simulink model "SecRwLtStZeroCtrl"  (R2018b)
settings: Solver=FixedStepDiscrete  StartTime=0.0  StopTime=10.0  RelTol=1e-3
undefined symbols (not defined in the file or in its folder): KeSMSuMdMotFinshdTm_Val, KeSMSuMdRetryTm1_Val, KeSMSuModeReqDurgTm_Val, KeSMSwSecRwLtStZeroEnTrigBitMask_Val
libraries: StCtrlLibBkRecln x1
settings Model: Creator=sn2xws  LastModifiedBy=sn55gm
settings Model: ModifiedHistory=|
  | 2024.5.6
  | 557 First Release
  | 2024.8.14 bitmask更换为port接口
settings DataIOCC: SaveFormat=StructureWithTime
settings OptimizationCC: DefaultParameterBehavior=Inlined  EnhancedBackFolding=on  PassReuseOutputArgsAs=Individual arguments  ZeroExternalMemoryAtStartup=off  ZeroInternalMemoryAtStartup=off  OptimizeBlockOrder=speed  DifferentSizesBufferReuse=on  OptimizationCustomize=off
settings DebuggingCC: ParameterTunabilityLossMsg=error
settings SFSimCC: MATLABDynamicMemAlloc=off
settings RTWCC: SystemTargetFile=autosar.tlc  GenCodeOnly=on  TemplateMakefile=ert_default_tmf  Description=AUTOSAR  GenerateReport=on  IncludeHyperlinkInReport=on  LaunchReport=on  GenerateTraceInfo=on  GenerateTraceReport=on  GenerateTraceReportSl=on  GenerateTraceReportSf=on  GenerateTraceReportEml=on
settings CodeAppCC: ForceParamTrailComments=on  IgnoreCustomStorageClasses=off  OperatorAnnotations=on  SimulinkDataObjDesc=on  SFDataObjDesc=on  InsertBlockDesc=on
settings STFCustomTargetCC: TargetLangStandard=C99 (ISO)  MultiwordLength=256  ParMdlRefBuildCompliant=on  CompOptLevelCompliant=on  IncludeMdlTerminateFcn=off  CombineOutputUpdateFcns=on  SuppressErrorStatus=on  ERTCustomFileBanners=on  SupportNonFinite=off  SupportComplex=off  SupportContinuousTime=off  SupportNonInlinedSFcns=off  RemoveResetFunc=on  MATLABClassNameForMDSCustomization=Simulink.SoftwareTarget.ERTCustomization  AutosarCompliant=on  UseToolchainInfoCompliant=on  LookupTableObjectStructAxisOrder=2,1,3,4,...  LUTObjectStructOrderEvenSpacing=Size,Table,Breakpoints  SystemTargetFile=autosar.tlc
settings ERTTargetCC: TargetLangStandard=C99 (ISO)  ConcurrentExecutionCompliant=off  IncludeMdlTerminateFcn=off  SuppressErrorStatus=on  SupportNonFinite=off  SupportComplex=off  ModelStepFunctionPrototypeControlCompliant=off  CPPClassGenCompliant=off  AutosarCompliant=on  LookupTableObjectStructAxisOrder=2,1,3,4,...  LUTObjectStructOrderEvenSpacing=Size,Table,Breakpoints  InlinedParameterPlacement=NonHierarchical  ERTCustomFileTemplate=example_file_process.tlc  ERTFilePackagingFormat=Compact

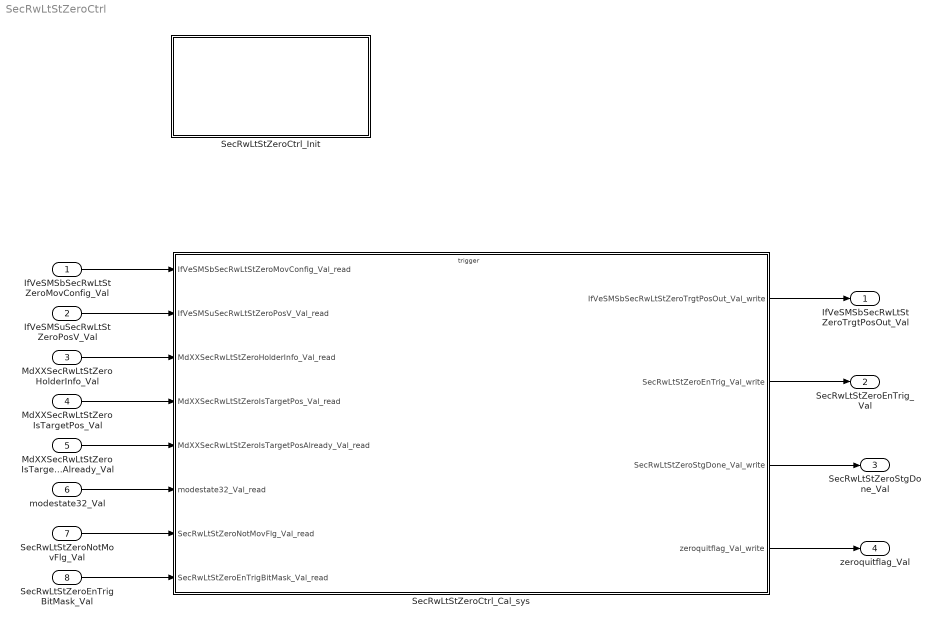
== system SecRwLtStZeroCtrl ==
  IfVeSMSbSecRwLtStZeroMovConfig_Val : Inport  OutDataTypeStr=boolean  PortDimensions=1
  IfVeSMSuSecRwLtStZeroPosV_Val : Inport  Port=2  OutDataTypeStr=boolean  PortDimensions=1
  MdXXSecRwLtStZeroHolderInfo_Val : Inport  Port=3  OutDataTypeStr=uint32  PortDimensions=1
  MdXXSecRwLtStZeroIsTargetPos_Val : Inport  Port=4  OutDataTypeStr=uint32  PortDimensions=1
  MdXXSecRwLtStZeroIsTargetPosAlready_Val : Inport  Port=5  OutDataTypeStr=uint32  PortDimensions=1
  modestate32_Val : Inport  Port=6  OutDataTypeStr=uint32  PortDimensions=1
  SecRwLtStZeroNotMovFlg_Val : Inport  Port=7  OutDataTypeStr=boolean  PortDimensions=1
  SecRwLtStZeroEnTrigBitMask_Val : Inport  Port=8  OutDataTypeStr=uint32  PortDimensions=1
  SecRwLtStZeroCtrl_Cal_sys : Subsystem
  SecRwLtStZeroCtrl_Init : Subsystem
  IfVeSMSbSecRwLtStZeroTrgtPosOut_Val : Outport  OutDataTypeStr=boolean  PortDimensions=1
  SecRwLtStZeroEnTrig_Val : Outport  Port=2  OutDataTypeStr=boolean  PortDimensions=1
  SecRwLtStZeroStgDone_Val : Outport  Port=3  OutDataTypeStr=boolean  PortDimensions=1
  zeroquitflag_Val : Outport  Port=4  OutDataTypeStr=boolean  PortDimensions=1
  wires:
  IfVeSMSbSecRwLtStZeroMovConfig_Val/1 -> SecRwLtStZeroCtrl_Cal_sys/1(IfVeSMSbSecRwLtStZeroMovConfig_Val_read)
  IfVeSMSuSecRwLtStZeroPosV_Val/1 -> SecRwLtStZeroCtrl_Cal_sys/2(IfVeSMSuSecRwLtStZeroPosV_Val_read)
  MdXXSecRwLtStZeroHolderInfo_Val/1 -> SecRwLtStZeroCtrl_Cal_sys/3(MdXXSecRwLtStZeroHolderInfo_Val_read)
  MdXXSecRwLtStZeroIsTargetPos_Val/1 -> SecRwLtStZeroCtrl_Cal_sys/4(MdXXSecRwLtStZeroIsTargetPos_Val_read)
  MdXXSecRwLtStZeroIsTargetPosAlready_Val/1 -> SecRwLtStZeroCtrl_Cal_sys/5(MdXXSecRwLtStZeroIsTargetPosAlready_Val_read)
  modestate32_Val/1 -> SecRwLtStZeroCtrl_Cal_sys/6(modestate32_Val_read)
  SecRwLtStZeroNotMovFlg_Val/1 -> SecRwLtStZeroCtrl_Cal_sys/7(SecRwLtStZeroNotMovFlg_Val_read)
  SecRwLtStZeroCtrl_Cal_sys/1(IfVeSMSbSecRwLtStZeroTrgtPosOut_Val_write) -> IfVeSMSbSecRwLtStZeroTrgtPosOut_Val/1
  SecRwLtStZeroCtrl_Cal_sys/2(SecRwLtStZeroEnTrig_Val_write) -> SecRwLtStZeroEnTrig_Val/1
  SecRwLtStZeroCtrl_Cal_sys/3(SecRwLtStZeroStgDone_Val_write) -> SecRwLtStZeroStgDone_Val/1
  SecRwLtStZeroEnTrigBitMask_Val/1 -> SecRwLtStZeroCtrl_Cal_sys/8(SecRwLtStZeroEnTrigBitMask_Val_read)
  SecRwLtStZeroCtrl_Cal_sys/4(zeroquitflag_Val_write) -> zeroquitflag_Val/1

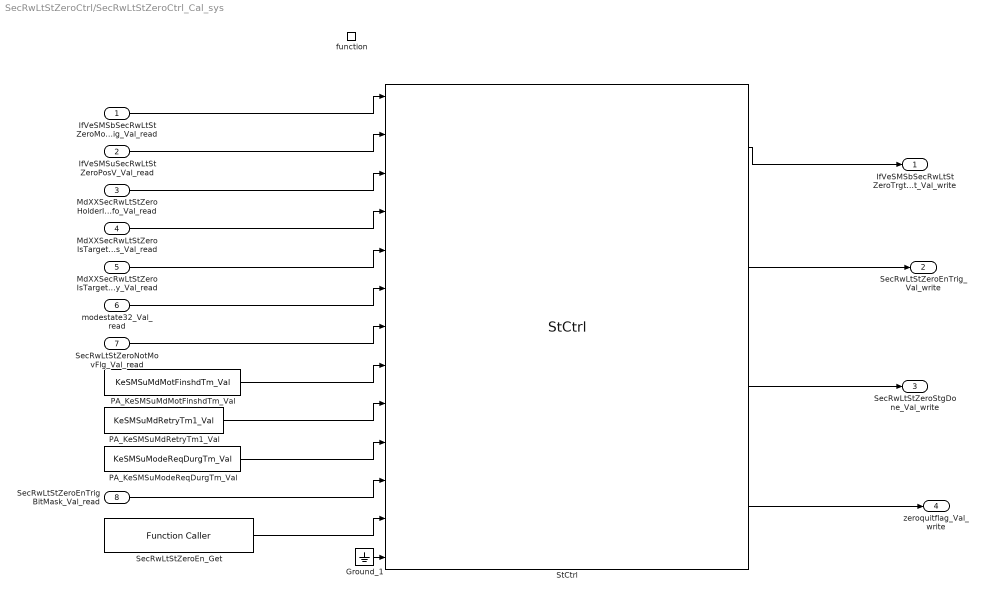
== system SecRwLtStZeroCtrl/SecRwLtStZeroCtrl_Cal_sys ==
  IfVeSMSbSecRwLtStZeroMovConfig_Val_read : Inport
  IfVeSMSuSecRwLtStZeroPosV_Val_read : Inport  Port=2
  MdXXSecRwLtStZeroHolderInfo_Val_read : Inport  Port=3
  MdXXSecRwLtStZeroIsTargetPos_Val_read : Inport  Port=4
  MdXXSecRwLtStZeroIsTargetPosAlready_Val_read : Inport  Port=5
  modestate32_Val_read : Inport  Port=6
  SecRwLtStZeroNotMovFlg_Val_read : Inport  Port=7
  SecRwLtStZeroEnTrigBitMask_Val_read : Inport  Port=8
  function : TriggerPort  TriggerType=function-call  IsSimulinkFunction=on  FunctionName=SecRwLtStZeroCtrl_Cal  VariantControl=(inherit)
  Ground_1 : Ground
  PA_KeSMSuMdMotFinshdTm_Val : Constant  Value=KeSMSuMdMotFinshdTm_Val
  PA_KeSMSuMdRetryTm1_Val : Constant  Value=KeSMSuMdRetryTm1_Val
  PA_KeSMSuModeReqDurgTm_Val : Constant  Value=KeSMSuModeReqDurgTm_Val
  SecRwLtStZeroEn_Get : FunctionCaller  FunctionPrototype=data = SecRwLtStZeroEn_Get()  OutputArgumentSpecifications=uint32(1)
  StCtrl : StCtrlLibBkRecln/StCtrl  SystemSampleTime=-1
  IfVeSMSbSecRwLtStZeroTrgtPosOut_Val_write : Outport
      settings: EnsureOutportIsVirtual=on
  SecRwLtStZeroEnTrig_Val_write : Outport  Port=2
      settings: EnsureOutportIsVirtual=on
  SecRwLtStZeroStgDone_Val_write : Outport  Port=3
      settings: EnsureOutportIsVirtual=on
  zeroquitflag_Val_write : Outport  Port=4
      settings: EnsureOutportIsVirtual=on
  wires:
  IfVeSMSbSecRwLtStZeroMovConfig_Val_read/1 -> StCtrl/1
  IfVeSMSuSecRwLtStZeroPosV_Val_read/1 -> StCtrl/2
  MdXXSecRwLtStZeroHolderInfo_Val_read/1 -> StCtrl/3
  MdXXSecRwLtStZeroIsTargetPos_Val_read/1 -> StCtrl/4
  MdXXSecRwLtStZeroIsTargetPosAlready_Val_read/1 -> StCtrl/5
  modestate32_Val_read/1 -> StCtrl/6
  SecRwLtStZeroNotMovFlg_Val_read/1 -> StCtrl/7
  PA_KeSMSuMdMotFinshdTm_Val/1 -> StCtrl/8
  PA_KeSMSuMdRetryTm1_Val/1 -> StCtrl/9
  PA_KeSMSuModeReqDurgTm_Val/1 -> StCtrl/10
  SecRwLtStZeroEnTrigBitMask_Val_read/1 -> StCtrl/11
  SecRwLtStZeroEn_Get/1 -> StCtrl/12
  StCtrl/1 -> IfVeSMSbSecRwLtStZeroTrgtPosOut_Val_write/1
  StCtrl/2 -> SecRwLtStZeroEnTrig_Val_write/1
  StCtrl/3 -> SecRwLtStZeroStgDone_Val_write/1
  Ground_1/1 -> StCtrl/13
  StCtrl/4 -> zeroquitflag_Val_write/1

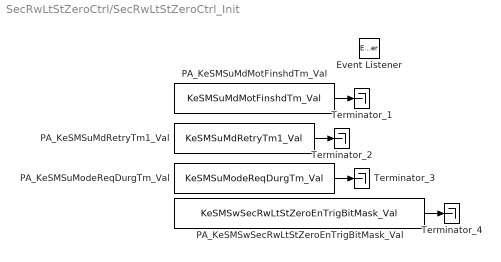
== system SecRwLtStZeroCtrl/SecRwLtStZeroCtrl_Init ==
  Event Listener : EventListener  EventName=reset
  PA_KeSMSuMdMotFinshdTm_Val : Constant  Value=KeSMSuMdMotFinshdTm_Val
  PA_KeSMSuMdRetryTm1_Val : Constant  Value=KeSMSuMdRetryTm1_Val
  PA_KeSMSuModeReqDurgTm_Val : Constant  Value=KeSMSuModeReqDurgTm_Val
  PA_KeSMSwSecRwLtStZeroEnTrigBitMask_Val : Constant  Value=KeSMSwSecRwLtStZeroEnTrigBitMask_Val
  Terminator_{1..4} (4 alike) : Terminator
  wires:
  PA_KeSMSuMdMotFinshdTm_Val/1 -> Terminator_1/1
  PA_KeSMSuMdRetryTm1_Val/1 -> Terminator_2/1
  PA_KeSMSuModeReqDurgTm_Val/1 -> Terminator_3/1
  PA_KeSMSwSecRwLtStZeroEnTrigBitMask_Val/1 -> Terminator_4/1
